simulink model "simple_SMC"  (R2022b)
settings: Solver=VariableStepAuto  StartTime=0.0  StopTime=30  RelTol=1e-3
settings Model: Creator=Adan Daniel  LastModifiedBy=Adan Daniel

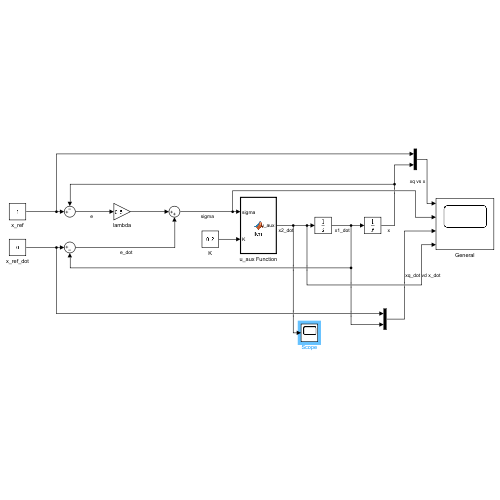
[thumbnail: Simulink's stored preview of the top-level diagram]
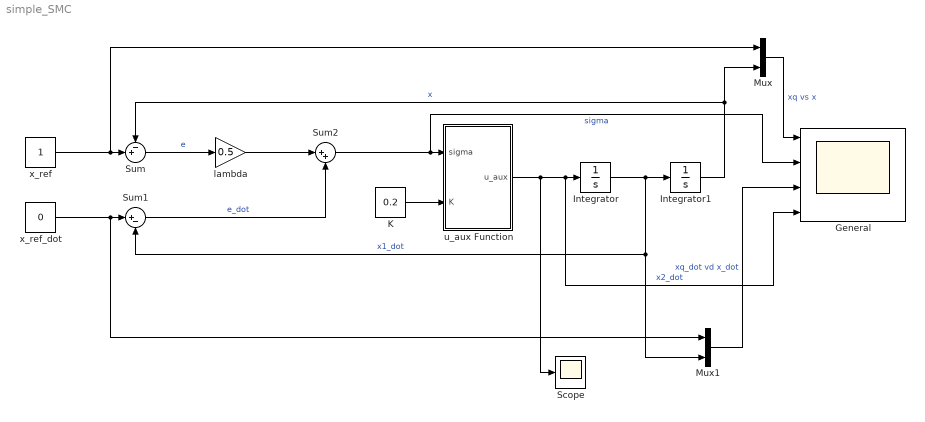
== system simple_SMC ==
  General : Scope  NumInputPorts=4
  Integrator : Integrator
  Integrator1 : Integrator
  K : Constant  Value=0.2
  Mux : Mux  Inputs=2
  Mux1 : Mux  Inputs=2
  Scope : Scope
  Sum : Sum  Inputs=-+|
  Sum1 : Sum  Inputs=|+-
  Sum2 : Sum  Inputs=|++
  lambda : Gain  Gain=0.5
  u_aux Function : MATLAB Function  TreatAsAtomicUnit=on
  x_ref : Constant
  x_ref_dot : Constant  Value=0
  wires:
  x_ref/1 -> Mux/1, Sum/2
  x_ref_dot/1 -> Mux1/1, Sum1/1
  Sum/1 -> lambda/1  "e"
  Sum1/1 -> Sum2/2  "e_dot"
  lambda/1 -> Sum2/1
  Sum2/1 -> General/2, u_aux Function/1(sigma)  "sigma"
  K/1 -> u_aux Function/2(K)
  u_aux Function/1(u_aux) -> Scope/1, General/4, Integrator/1  "x2_dot"
  Integrator/1 -> Mux1/2, Sum1/2, Integrator1/1  "x1_dot"
  Integrator1/1 -> Mux/2, Sum/1  "x"
  Mux/1 -> General/1  "xq vs x"
  Mux1/1 -> General/3  "xq_dot vd x_dot"

== matlab function simple_SMC/u_aux Function ==
  data: sigma input; u_aux output; K input
function u_aux = fcn(sigma, K)

u_aux = K * (abs(sigma))^(0.05) *sign(sigma);
